simulink model "windturb"  (R2021a)
settings: Solver=VariableStepAuto  StartTime=0.0  StopTime=24*60*60  RelTol=1e-3
values from neighbouring files (symbols this model uses):
  time = [1 1.0167 1.0333 1.05 1.0667 1.0833 1.1 1.1167 1.1333 1.15 1.1667 1.1833 ... (1381 elements, 1x1381)]    [time.mat]    (also in time2.mat = [1 1.0167 1.0333 1.05 1.0667 1.0833 1.1 1.1167 1.1333 1.15 1)
  wind = [9 9 9 9 9 9 9 9 9 9 9 9 ... (1381 elements, 1x1381)]    [wind_data.mat]
settings Model: Creator=lassenielsen  LastModifiedBy=cm

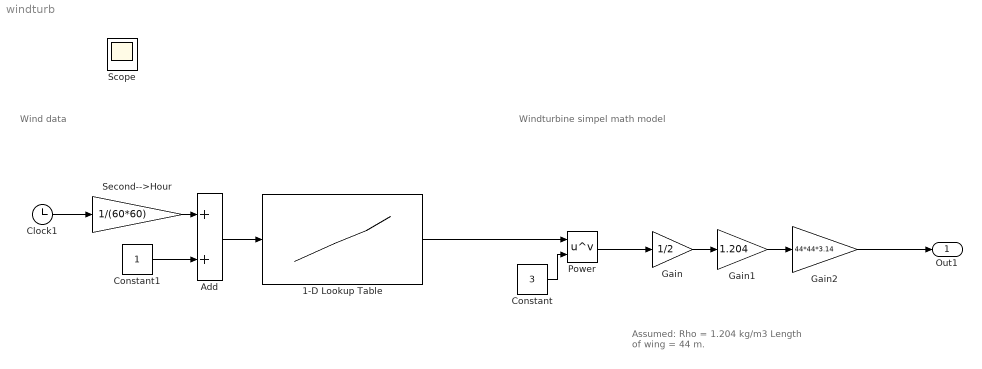
== system windturb ==
  note: Wind data
  note: Assumed:
      | Rho = 1.204 kg/m3
      | Length of wing = 44 m.
  note: Windturbine simpel math model
  1-D Lookup Table : Lookup_n-D  NumberOfTableDimensions=1  BreakpointsForDimension1=time  BeginIndexSearchUsingPreviousIndexResult=on  Table=wind  ExtrapMethod=Clip  UseLastTableValue=on  InternalRulePriority=Speed  RndMeth=Simplest  InputSameDT=on
  Add : Sum
  Clock1 : Clock
  Constant : Constant  Value=3
  Constant1 : Constant
  Gain : Gain  Gain=1/2
  Gain1 : Gain  Gain=1.204
  Gain2 : Gain  Gain=44*44*3.14
  Power : Math  Operator=pow  SaturateOnIntegerOverflow=on
  Second-->Hour : Gain  Gain=1/(60*60)
  Out1 : Outport
  Scope : Scope
  wires:
  Second-->Hour/1 -> Add/1
  Add/1 -> 1-D Lookup Table/1
  Clock1/1 -> Second-->Hour/1
  Constant1/1 -> Add/2
  1-D Lookup Table/1 -> Power/1
  Constant/1 -> Power/2
  Power/1 -> Gain/1
  Gain/1 -> Gain1/1
  Gain1/1 -> Gain2/1
  Gain2/1 -> Out1/1
